simulink model "CognitiveRadio"  (Simulink 7.7)
settings: Solver=ode45  StartTime=0.0  StopTime=10.0  RelTol=1e-3
undefined symbols (not defined in the file or in its folder): Fs, get, sided, Two
libraries: commrandsrc2 x5, commanapbnd3 x5, dspsnks4 x1
settings Model: Creator=pc7  LastModifiedBy=Saifur
settings DebuggingCC: StrictBusMsg=Warning

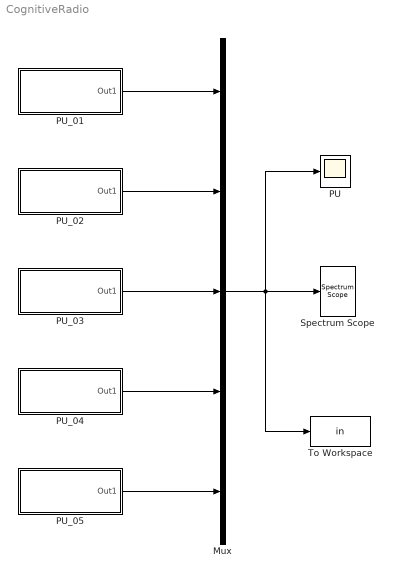
== system CognitiveRadio ==
  Mux : Mux  Inputs=5
  PU : Scope
      settings: SaveName=ScopeData10
  PU_01 : Subsystem
  PU_02 : Subsystem
  PU_03 : Subsystem
  PU_04 : Subsystem
  PU_05 : Subsystem
  Spectrum Scope : dspsnks4/Spectrum Scope  SystemSampleTime=-1  ScopeProperties=on  Domain=Frequency  HorizSpan=1  UseBuffer=on  BufferSize=128  Overlap=0  TreatMby1Signals=M channels  inpFftLenInherit=on  FFTlength=1024  numAvg=5  DisplayProperties=off  AxisGrid=on  Memory=off  FrameNumber=off  AxisLegend=off  AxisZoom=off  OpenScopeAtSimStart=on  OpenScopeImmediately=off  FigPos=get(0,'defaultfigureposition')  AxisProperties=off  XUnits=Hertz  XRange=Two-sided ((-Fs/2...Fs/2])  XDisplay=0  InheritXIncr=on  XIncr=1.0  XLabel=Samples  XLimit=Auto  YUnits=dBW/Hertz  XMax=1  XMin=0  YLabel=Magnitude-squared, dB  LineProperties=off  LineDisables=off  LineStyles=-|--|:  LineMarkers=|||o|*  wintypeSpecScope=Hamming  RsSpecScope=50  betaSpecScope=5  winsampSpecScope=Periodic  XAxisParamsVer=6.9  isFrameUpgraded=on
      settings: YMin=-30  YMax=30
  To Workspace : ToWorkspace  VariableName=in  SampleTime=-1  SaveFormat=Array
  wires:
  PU_01/1(Out1) -> Mux/1
  PU_02/1(Out1) -> Mux/2
  PU_03/1(Out1) -> Mux/3
  PU_04/1(Out1) -> Mux/4
  PU_05/1(Out1) -> Mux/5
  Mux/1 -> Spectrum Scope/1, PU/1, To Workspace/1

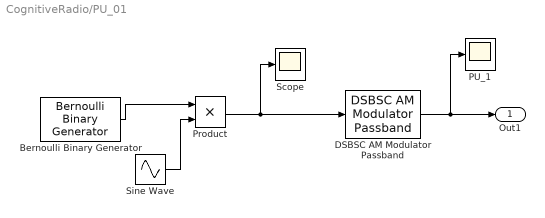
== system CognitiveRadio/PU_01 ==
  Bernoulli Binary Generator : commrandsrc2/Bernoulli Binary Generator  SystemSampleTime=-1  P=0.5  seed=61  Ts=100  frameBased=off  sampPerFrame=1  orient=off  outDataType=double
  DSBSC AM Modulator Passband : commanapbnd3/DSBSC AM Modulator Passband  SystemSampleTime=-1  Fc=12000  Ph=45
  PU_1 : Scope
  Product : Product  RndMeth=Zero
  Scope : Scope
  Sine Wave : Sin  Amplitude=5  Frequency=4340  SampleTime=2
  Out1 : Outport
  wires:
  Bernoulli Binary Generator/1 -> Product/1
  Sine Wave/1 -> Product/2
  Product/1 -> Scope/1, DSBSC AM Modulator Passband/1
  DSBSC AM Modulator Passband/1 -> PU_1/1, Out1/1

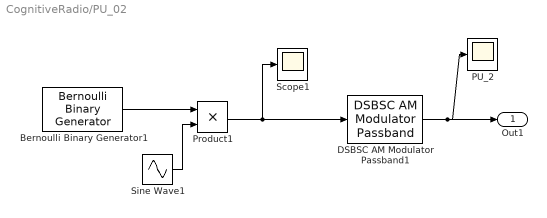
== system CognitiveRadio/PU_02 ==
  Bernoulli Binary Generator1 : commrandsrc2/Bernoulli Binary Generator  SystemSampleTime=-1  P=0.5  seed=61  Ts=100  frameBased=off  sampPerFrame=1  orient=off  outDataType=double
  DSBSC AM Modulator Passband1 : commanapbnd3/DSBSC AM Modulator Passband  SystemSampleTime=-1  Fc=13000  Ph=0
  PU_2 : Scope
      settings: SaveName=ScopeData2
  Product1 : Product  RndMeth=Zero
  Scope1 : Scope
      settings: SaveName=ScopeData3
  Sine Wave1 : Sin  Amplitude=5  Frequency=4968  SampleTime=2
  Out1 : Outport
  wires:
  Bernoulli Binary Generator1/1 -> Product1/1
  Sine Wave1/1 -> Product1/2
  Product1/1 -> Scope1/1, DSBSC AM Modulator Passband1/1
  DSBSC AM Modulator Passband1/1 -> PU_2/1, Out1/1

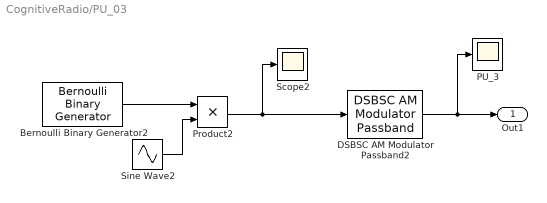
== system CognitiveRadio/PU_03 ==
  Bernoulli Binary Generator2 : commrandsrc2/Bernoulli Binary Generator  SystemSampleTime=-1  P=0.5  seed=61  Ts=100  frameBased=off  sampPerFrame=1  orient=off  outDataType=double
  DSBSC AM Modulator Passband2 : commanapbnd3/DSBSC AM Modulator Passband  SystemSampleTime=-1  Fc=14000  Ph=0
  PU_3 : Scope
      settings: SaveName=ScopeData4
  Product2 : Product  RndMeth=Zero
  Scope2 : Scope
      settings: SaveName=ScopeData5
  Sine Wave2 : Sin  Amplitude=5  Frequency=628  SampleTime=2
  Out1 : Outport
  wires:
  Bernoulli Binary Generator2/1 -> Product2/1
  Sine Wave2/1 -> Product2/2
  Product2/1 -> Scope2/1, DSBSC AM Modulator Passband2/1
  DSBSC AM Modulator Passband2/1 -> PU_3/1, Out1/1

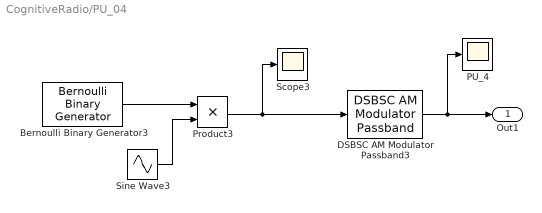
== system CognitiveRadio/PU_04 ==
  Bernoulli Binary Generator3 : commrandsrc2/Bernoulli Binary Generator  SystemSampleTime=-1  P=0.5  seed=61  Ts=1  frameBased=off  sampPerFrame=100  orient=off  outDataType=double
  DSBSC AM Modulator Passband3 : commanapbnd3/DSBSC AM Modulator Passband  SystemSampleTime=-1  Fc=15000  Ph=0
  PU_4 : Scope
      settings: SaveName=ScopeData6
  Product3 : Product  RndMeth=Zero
  Scope3 : Scope
      settings: SaveName=ScopeData7
  Sine Wave3 : Sin  Amplitude=5  Frequency=1256  SampleTime=2
  Out1 : Outport
  wires:
  Bernoulli Binary Generator3/1 -> Product3/1
  Product3/1 -> Scope3/1, DSBSC AM Modulator Passband3/1
  DSBSC AM Modulator Passband3/1 -> PU_4/1, Out1/1
  Sine Wave3/1 -> Product3/2

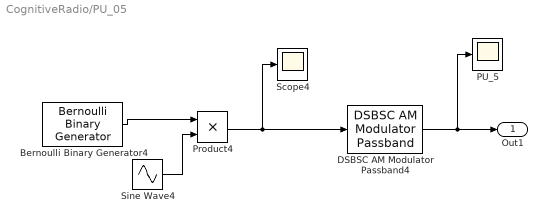
== system CognitiveRadio/PU_05 ==
  Bernoulli Binary Generator4 : commrandsrc2/Bernoulli Binary Generator  SystemSampleTime=-1  P=0.5  seed=61  Ts=100  frameBased=off  sampPerFrame=1  orient=off  outDataType=double
  DSBSC AM Modulator Passband4 : commanapbnd3/DSBSC AM Modulator Passband  SystemSampleTime=-1  Fc=16000  Ph=0
  PU_5 : Scope
      settings: SaveName=ScopeData8
  Product4 : Product  RndMeth=Zero
  Scope4 : Scope
      settings: SaveName=ScopeData9
  Sine Wave4 : Sin  Amplitude=5  Frequency=3712  SampleTime=2
  Out1 : Outport
  wires:
  Bernoulli Binary Generator4/1 -> Product4/1
  Sine Wave4/1 -> Product4/2
  Product4/1 -> Scope4/1, DSBSC AM Modulator Passband4/1
  DSBSC AM Modulator Passband4/1 -> PU_5/1, Out1/1
